simulink model "DSM3"  (R2020a)
settings: Solver=VariableStepAuto  StartTime=0.0  StopTime=0.6  RelTol=1e-3
settings Model: Creator=bzhan  LastModifiedBy=bzhan

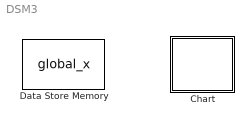
== system DSM3 ==
  Chart : Stateflow chart  TreatAsAtomicUnit=on
  Data Store Memory : DataStoreMemory  DataStoreName=global_x  ReadBeforeWriteMsg=warning  WriteAfterWriteMsg=warning  WriteAfterReadMsg=warning  InitialValue=[1 2]  ShowAdditionalParam=off  OutDataTypeStr=int32

== stateflow chart DSM3/Chart ==
  settings: updateMethod=DISCRETE  sampleTime=0.1
  state A
  state B
  (default) -> A : {v=0;}
  A -> B : {v=global_x(1);global_x(1)=global_x(2)+v;f()}
  B -> A : {v=global_x(2);global_x(2)=global_x(1)+v;f()}
  data: global_x data_store_memory; v local int32
  function f:
    | function f
    |   fprintf("%d %d\n", global_x(1), global_x(2));
